simulink model "test_capt"  (Simulink 7.3)
settings: Solver=ode45  StartTime=0  StopTime=2500  RelTol=1e-3
undefined symbols (not defined in the file): capt_4x, isi_correlator_lib
libraries: xbsIndex_r4 x13, xps_library x4, casper_library x2
settings Model: Creator=wjm  LastModifiedBy=wjm

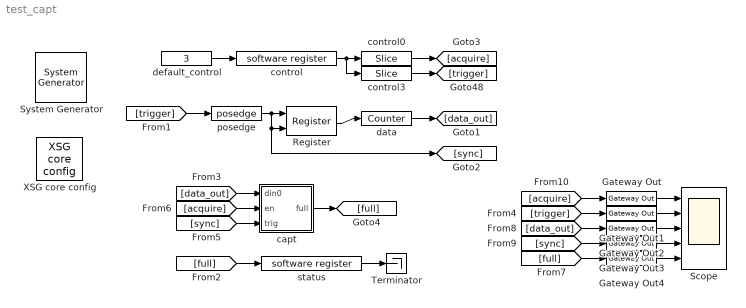
== system test_capt ==
  " System Generator" : xbsIndex_r4/ System Generator  Tag=genX  SystemSampleTime=-1  xilinxfamily=virtex5  part=xc5vsx95t  speed=-1  package=ff1136  synthesis_tool=XST  clock_wrapper=Clock Enables  directory=./test_capt/sysgen  testbench=off  simulink_period=1  sysclk_period=5  dcm_input_clock_period=100  incr_netlist=off  trim_vbits=Everywhere in SubSystem  dbl_ovrd=According to Block Masks  core_generation=According to Block Masks  run_coregen=off  deprecated_control=off  eval_field=0  block_type=sysgen
      settings: block_version=11.3
  Gateway Out{,1..4} (5 alike) : xbsIndex_r4/Gateway Out  hdl_port=on  timing_constraint=None  locs_specified=off  LOCs={}  block_type=gatewayout
      settings: infoedit="Gateway out block.  Converts Xilinx fixed point inputs into ouputs of type Simulink integer, double, or fixed point.<br><br>Hardware notes:  In hardware these blocks become top level output ports or are discarded, depending on how they are configured."  block_version=11.3
  Register : xbsIndex_r4/Register  init=0  rst=off  en=on  dbl_ovrd=off  block_type=register
      settings: block_version=11.3
  Scope : Scope  NumInputPorts=5
      settings: YMin=-5~-5~-5~-5~-5  YMax=5~5~5~5~5
  Terminator : Terminator
  XSG core config : xps_library/XSG core config  Tag=xps:xsg  SystemSampleTime=-1  hw_sys=ROACH:sx95t  ibob_linux=off  clk_src=sys_clk2x  iBOB_clk_src=sys_clk  BEE2_ctrl_clk_src=sys_clk  BEE2_usr_clk_src=sys_clk  ROACH_clk_src=sys_clk2x  CORR_clk_src=sys_clk  gpio_clk_io_group=iBOB:sma  gpio_clk_bit_index=0  clk_rate=200  sample_period=1  synthesis_tool=XST  mpc_type=powerpc440_ext
  capt : Subsystem  AncestorBlock=isi_correlator_lib/capt_4x
  control : xps_library/software register  Tag=xps:sw_reg  SystemSampleTime=-1  io_dir=From Processor  arith_type=Unsigned  bitwidth=32  bin_pt=0  sample_period=1  gw_name=test_capt_control_user_data_out
      link override corr_3ghz_10_1_corr_id_user_data_out: arith_type=Unsigned  n_bits=32  bin_pt=0  period=1
      link override corr_3ghz_10_1_exp_corr_id_user_data_out: arith_type=Unsigned  n_bits=32  bin_pt=0  period=1
      link override isi_corr_eq_coeff_user_data_out: arith_type=Unsigned  n_bits=32  bin_pt=0  period=1
      link override isi_correlator_control_user_data_out: arith_type=Unsigned  n_bits=32  bin_pt=0  period=1
      link override isi_correlator_cropped_control_user_data_out: arith_type=Unsigned  n_bits=32  bin_pt=0  period=1
      link override isi_correlator_eq_coeff_user_data_out: arith_type=Unsigned  n_bits=32  bin_pt=0  period=1
      link override isi_spectrometer_control_user_data_out: arith_type=Unsigned  n_bits=32  bin_pt=0  period=1
      link override isi_spectrometer_cropped_control_user_data_out: arith_type=Unsigned  n_bits=32  bin_pt=0  period=1
      link override isi_spectrometer_with_pfb_control_user_data_out: arith_type=Unsigned  n_bits=32  bin_pt=0  period=1
      link override roach_spectrometer_control_user_data_out: arith_type=Unsigned  n_bits=32  bin_pt=0  period=1
      link override test_link_mux_demux_control_user_data_out: arith_type=Unsigned  n_bits=32  bin_pt=0  period=1
  control0 : xbsIndex_r4/Slice  nbits=1  boolean_output=on  mode=Lower Bit Location + Width  bit1=0  base1=MSB of Input  bit0=0  base0=LSB of Input  dbl_ovrd=off  block_type=slice
      settings: infoedit="Extracts a given range of bits from each input sample and presents it at the output.  The output type is ordinarily unsigned with binary point at zero, but can be Boolean when the slice is one bit wide.<P><P>Hardware notes: In hardware this block costs nothing."  block_version=10.1.3
  control3 : xbsIndex_r4/Slice  nbits=1  boolean_output=on  mode=Lower Bit Location + Width  bit1=0  base1=MSB of Input  bit0=1  base0=LSB of Input  dbl_ovrd=off  block_type=slice
      settings: block_version=10.1.3
  data : xbsIndex_r4/Counter  cnt_type=Free Running  cnt_to=Inf  operation=Up  start_count=0  cnt_by_val=1  arith_type=Unsigned  n_bits=32  bin_pt=0  load_pin=off  rst=off  en=on  explicit_period=on  period=1  dbl_ovrd=off  use_behavioral_HDL=off  implementation=Fabric  block_type=counter
      settings: block_version=11.3
  default_control : Constant  Value=3  OutDataType=sfix(16)  OutScaling=2^0  SampleTime=1
  posedge : casper_library/Misc/posedge  Tag=Rising Edge Detector  SystemSampleTime=-1
  status : xps_library/software register  Tag=xps:sw_reg  SystemSampleTime=-1  io_dir=To Processor  arith_type=Unsigned  bitwidth=32  bin_pt=0  sample_period=1  gw_name=test_capt_status_user_data_in
      link override corr_3ghz_10_1_corr_id_user_data_out: arith_type=Unsigned  n_bits=32  bin_pt=0  period=1
      link override corr_3ghz_10_1_exp_corr_id_user_data_out: arith_type=Unsigned  n_bits=32  bin_pt=0  period=1
      link override isi_corr_eq_coeff_user_data_out: arith_type=Unsigned  n_bits=32  bin_pt=0  period=1
      link override isi_correlator_control_user_data_out: arith_type=Unsigned  n_bits=32  bin_pt=0  period=1
      link override isi_correlator_cropped_control_user_data_out: arith_type=Unsigned  n_bits=32  bin_pt=0  period=1
      link override isi_correlator_eq_coeff_user_data_out: arith_type=Unsigned  n_bits=32  bin_pt=0  period=1
      link override isi_spectrometer_control_user_data_out: arith_type=Unsigned  n_bits=32  bin_pt=0  period=1
      link override isi_spectrometer_cropped_control_user_data_out: arith_type=Unsigned  n_bits=32  bin_pt=0  period=1
      link override isi_spectrometer_with_pfb_control_user_data_out: arith_type=Unsigned  n_bits=32  bin_pt=0  period=1
      link override roach_spectrometer_control_user_data_out: arith_type=Unsigned  n_bits=32  bin_pt=0  period=1
      link override test_link_mux_demux_control_user_data_out: arith_type=Unsigned  n_bits=32  bin_pt=0  period=1
  wires:
  control/1 -> control0/1, control3/1
  default_control/1 -> control/1
  control0/1 -> [acquire]
  [data_out] -> capt/1(din0)
  control3/1 -> [trigger]
  [acquire] -> capt/2(en)
  data/1 -> [data_out]
  [sync] -> capt/3(trig)
  [trigger] -> posedge/1
  capt/1(full) -> [full]
  [full] -> status/1
  status/1 -> Terminator/1
  [acquire] -> Gateway Out/1
  [trigger] -> Gateway Out1/1
  [data_out] -> Gateway Out2/1
  [sync] -> Gateway Out3/1
  [full] -> Gateway Out4/1
  Gateway Out/1 -> Scope/1
  Gateway Out1/1 -> Scope/2
  Gateway Out2/1 -> Scope/3
  Gateway Out3/1 -> Scope/4
  Gateway Out4/1 -> Scope/5
  Register/1 -> data/1
  posedge/1 -> Register/1, Register/2, [sync]

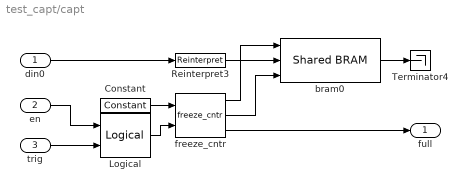
== system test_capt/capt ==
  din0 : Inport  OutDataType=sfix(16)  OutScaling=2^0
  en : Inport  Port=2  OutDataType=sfix(16)  OutScaling=2^0
  trig : Inport  Port=3  OutDataType=sfix(16)  OutScaling=2^0
  Constant : xbsIndex_r4/Constant  arith_type=Boolean  const=1  n_bits=1  bin_pt=0  explicit_period=on  period=1  equ=P=C  opselect=C  inp2=PCIN>>17  opr=+  inp1=P  carry=CIN  dbl_ovrd=off  block_type=constant
      settings: block_version=10.1.1
  Logical : xbsIndex_r4/Logical  logical_function=AND  inputs=2  en=off  latency=0  precision=Full  arith_type=Unsigned  n_bits=1  bin_pt=0  align_bp=on  dbl_ovrd=off  block_type=logical
      settings: block_version=10.1.1
  Reinterpret3 : xbsIndex_r4/Reinterpret  force_arith_type=on  arith_type=Unsigned  force_bin_pt=on  bin_pt=0  block_type=reinterpret
      settings: infoedit="Changes signal type without altering the binary representation.   You can changed the signal between signed and unsigned, and relocate the binary point.<P><P>Hardware notes: In hardware this block costs nothing.<P><P>Example:  Suppose the input is 6 bits wide, signed, with 2 fractional bits, and the output is forced to unsigned with 0 fractional bits.  Then an input of -2.0 (1110.00 in binary 2's complement) becomes an output of 56 (111000 in binary)."  block_version=10.1.1
  Terminator4 : Terminator
  bram0 : xps_library/Shared BRAM  Tag=xps:bram  SystemSampleTime=-1  arith_type=Unsigned  addr_width=11  data_width=32  data_bin_pt=0  init_vals=0  sample_rate=1
  freeze_cntr : casper_library/Misc/freeze_cntr  SystemSampleTime=-1  CounterBits=11
  full : Outport  OutDataType=fixdt(1, 16)  OutScaling=2^0
  wires:
  freeze_cntr/1 -> bram0/1
  freeze_cntr/2 -> bram0/3
  freeze_cntr/3 -> full/1
  Reinterpret3/1 -> bram0/2
  din0/1 -> Reinterpret3/1
  bram0/1 -> Terminator4/1
  Logical/1 -> freeze_cntr/2
  Constant/1 -> freeze_cntr/1
  en/1 -> Logical/1
  trig/1 -> Logical/2
